simulink model "FirstCode_HardwareHarness"  (R2014b)
settings: Solver=FixedStepDiscrete  StartTime=0.0  StopTime=10  RelTol=1e-3
PostLoadFcn:
  | c2000demoscallback(1)
undefined symbols (not defined in the file or in its folder): CR, serial
libraries: c2803xlib x2, instrumentlib x2, simulink x1, c280xlib x1
settings Model: Creator=The MathWorks Inc.  LastModifiedBy=Nathan
settings DataIOCC: SignalLoggingSaveFormat=ModelDataLogs  SaveOutput=off  SaveTime=off
settings OptimizationCC: ExpressionDepthLimit=2147483647  InitFltsAndDblsToZero=on  OptimizeModelRefInitCode=on  LifeSpan=Inf  MaxStackSize=64
settings DebuggingCC: UnderspecifiedInitializationDetection=Classic  MergeDetectMultiDrivingBlocksExec=none  SignalResolutionControl=TryResolveAllWithWarning  SolverPrmCheckMsg=none  InheritedTsInSrcMsg=none  MultiTaskDSMMsg=warning  MultiTaskCondExecSysMsg=none  FcnCallInpInsideContextMsg=UseLocalSettings  StateNameClashWarn=warning
settings HardwareCC: ProdBitPerChar=16  ProdBitPerInt=16  ProdBitPerPointer=16  ProdLargestAtomicInteger=Integer  ProdIntDivRoundTo=Zero  ProdEndianess=LittleEndian  ProdWordSize=16  ProdHWDeviceType=Texas Instruments->C2000  TargetBitPerChar=16  TargetBitPerInt=16  TargetBitPerPointer=16  TargetLargestAtomicInteger=Integer  TargetIntDivRoundTo=Zero  TargetEndianess=LittleEndian  TargetWordSize=16  TargetHWDeviceType=Texas Instruments->C2000
settings RTWCC: SystemTargetFile=ert.tlc  TemplateMakefile=ert_default_tmf  PostCodeGenCommand=; ;codertarget.postCodeGenHookCommand(h)  Description=Embedded Coder  GenerateReport=on  ProcessScript=ert_make_rtw_hook  Toolchain=Texas Instruments Code Composer Studio v5 (C2000)  BuildConfiguration=Faster Runs  IncludeHyperlinkInReport=on  PortableWordSizes=on  CodeExecutionProfiling=on  CodeProfilingInstrumentation=on
settings CodeAppCC: IgnoreCustomStorageClasses=off  CustomSymbolStrType=$N$R$M  InternalIdentifier=Classic

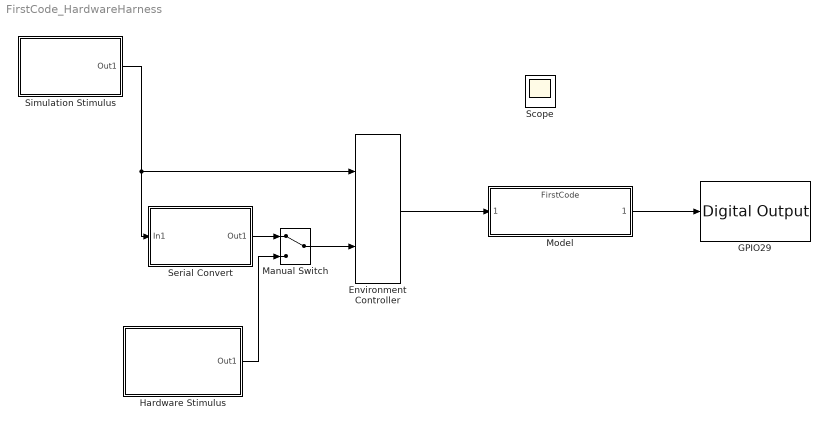
== system FirstCode_HardwareHarness ==
  Environment Controller : simulink/Signal Routing/Environment Controller
  GPIO29 : c2803xlib/Digital Output  GPIO_Number=GPIO24~GPIO31  GPIO_Bit0=off  GPIO_BIT0_Toggle=off  GPIO_Bit1=off  GPIO_BIT1_Toggle=off  GPIO_Bit2=off  GPIO_BIT2_Toggle=off  GPIO_Bit3=off  GPIO_BIT3_Toggle=off  GPIO_Bit4=off  GPIO_BIT4_Toggle=off  GPIO_Bit5=on  GPIO_BIT5_Toggle=off  GPIO_Bit6=off  GPIO_BIT6_Toggle=on  GPIO_Bit7=off  GPIO_BIT7_Toggle=off
  Hardware Stimulus : Subsystem
  Manual Switch : ManualSwitch
  Model : ModelReference  ModelNameDialog=FirstCode.slx  SimulationMode=Normal  ModelReferenceVersion=1.78  CopyOfModelName=FirstCode.slx  DefaultDataLogging=on
  Scope : Scope
      settings: Floating=on
  Serial Convert : Subsystem
  Simulation Stimulus : Subsystem
  wires:
  Environment Controller/1 -> Model/1
  Model/1 -> GPIO29/1
  Simulation Stimulus/1(Out1) -> Environment Controller/1, Serial Convert/1(In1)
  Hardware Stimulus/1(Out1) -> Manual Switch/2
  Manual Switch/1 -> Environment Controller/2
  Serial Convert/1(Out1) -> Manual Switch/1

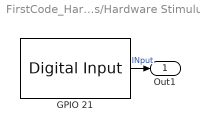
== system FirstCode_HardwareHarness/Hardware Stimulus ==
  "GPIO 21 " : c2803xlib/Digital Input  GPIO_Number=GPIO16~GPIO23  GPIO_Bit0=off  GPIO_Bit1=off  GPIO_Bit2=off  GPIO_Bit3=off  GPIO_Bit4=off  GPIO_Bit5=on  GPIO_Bit6=off  GPIO_Bit7=off  sampleTime=0.1  dataType=auto  GPIO_Bit0_Qualification=Sync to SYSCLKOUT  GPIO_Bit1_Qualification=Sync to SYSCLKOUT  GPIO_Bit2_Qualification=Sync to SYSCLKOUT  GPIO_Bit3_Qualification=Sync to SYSCLKOUT  GPIO_Bit4_Qualification=Sync to SYSCLKOUT  GPIO_Bit5_Qualification=Sync to SYSCLKOUT  GPIO_Bit6_Qualification=Sync to SYSCLKOUT  GPIO_Bit7_Qualification=Sync to SYSCLKOUT  Qualification_Period=-1
  Out1 : Outport
  wires:
  "GPIO 21 "/1 -> Out1/1  "INput"

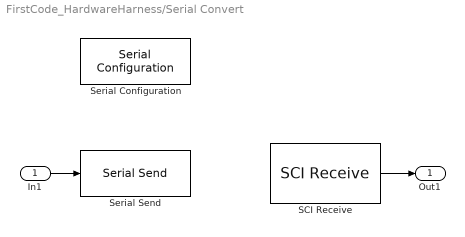
== system FirstCode_HardwareHarness/Serial Convert ==
  In1 : Inport
  SCI Receive : c280xlib/SCI Receive  sciModule=A  dataHead='S'  dataTail='\r'  dataType=uint8  dataDim=1  initValue=0  errOption=Output the last received value  errValue=0  sampleTime=0.1  outputStatus=off  postInterrupt=off  numFifo=0
  Serial Configuration : instrumentlib/Serial Configuration  Priority=-200000  ComPortMenu=COM11  ComPort=COM11  ObjConstructor=serial('COM11');  BaudRate=9600  DataBits=8  Parity=none  StopBits=1  FlowControl=none  Timeout=10  ByteOrder=LittleEndian
  Serial Send : instrumentlib/Serial Send  ComPortMenu=COM11  ComPort=COM11  ObjConstructor=serial('COM11');  Header='S'  Terminator=CR ('\r')  EnableBlockingMode=on
  Out1 : Outport
  wires:
  In1/1 -> Serial Send/1
  SCI Receive/1 -> Out1/1

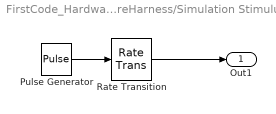
== system FirstCode_HardwareHarness/Simulation Stimulus ==
  Pulse Generator : DiscretePulseGenerator  PulseType=Time based  Period=1  PulseWidth=50
  Rate Transition : RateTransition  OutPortSampleTime=0.1
  Out1 : Outport
  wires:
  Pulse Generator/1 -> Rate Transition/1
  Rate Transition/1 -> Out1/1
